simulink model "pv_and_batt"  (Simulink 7.8)
settings: Solver=ode45  StartTime=0.0  StopTime=10.0  RelTol=1e-3
values from neighbouring files (symbols this model uses):
  f = 60    [global_parameters.m]
  PLL_time_step = Ts    (= 8e-05)    [global_parameters.m]
  Td_es_min = Ts    (= 8e-05)    [global_parameters.m]
  Tds = Ts    (= 8e-05)    [global_parameters.m]
  Ts = 80e-6    (= 8e-05)    [global_parameters.m]    (also in scopeBuffer.m)
undefined symbols (not defined in the file or in its folder): batt_esr, C, D, DiscIntNeverNeededParam, I_ki, I_kp, Iac_max, Id_at_max, Iq_at_max, L, PLL_Ki, PLL_Kp, Roff, Vdc_max
libraries: powerlib x38, simulink x17, simulink_extras x6, cstextras x6, powerlib_extras x2, rtlab x1
(part 1 of 2)
settings Model: Creator=re25624  LastModifiedBy=ma25949

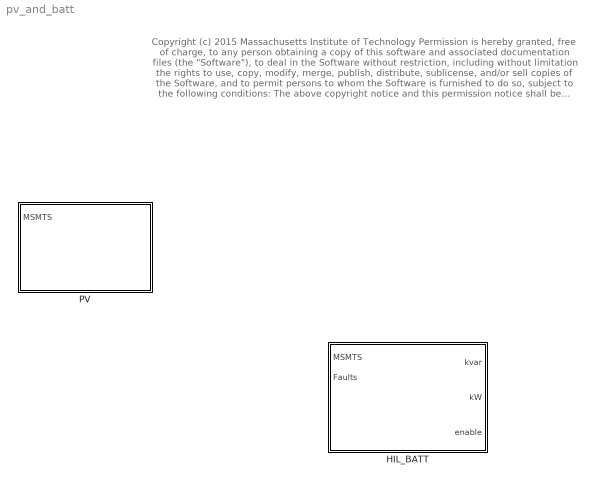
== system pv_and_batt ==
  note: Copyright (c) 2015 Massachusetts Institute of Technology
      | Permission is hereby granted, free of charge, to any person obtaining a copy of this software and associated documentation files (the "Software"), to deal in the Software without restriction, including without limitation the rights to use, copy, modify, merge, publish, distribute, sublicense, and/or sell copies of the Software, and to permit persons to whom the Software is furnished to do so, subject to the following conditions:
      |
      | The above copyright notice and this permission notice shall be included in all copies or substantial portions of the Software.
      |
      | THE SOFTWARE IS PROVIDED "AS IS", WITHOUT WARRANTY OF ANY KIND, EXPRESS OR IMPLIED, INCLUDING BUT NOT LIMITED TO THE WARRANTIES OF MERCHANTABILITY, FITNESS FOR A PARTICULAR PURPOSE AND NONINFRINGEMENT. IN NO EVENT SHALL THE AUTHORS OR COPYRIGHT HOLDERS BE LIABLE FOR ANY CLAIM,
      | DAMAGES OR OTHER LIABILITY, WHETHER IN AN ACTION OF CONTRACT, TORT OR OTHERWISE, ARISING FROM, OUT OF OR IN CONNECTION WITH THE SOFTWARE OR THE USE OR OTHER DEALINGS IN THE SOFTWARE.
  HIL_BATT : Subsystem
  PV : Subsystem

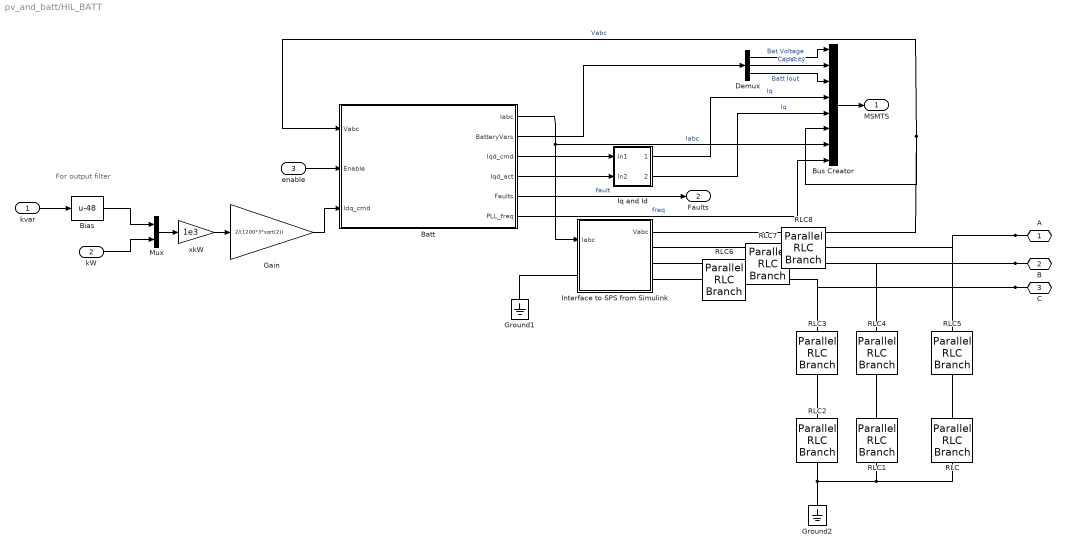
== system pv_and_batt/HIL_BATT ==
  note: For output filter
  kvar : Inport
  kW : Inport  Port=2
  enable : Inport  Port=3
  Batt : Subsystem  mask(Battery Energy Storage System with AC inverter and Droop Control){max_power=4e6, batt_kWh=5000, VacRMS=1200, Vdc_nom=4000}
      mask prompts: max_power "Peak Power (W)"; batt_kWh "Capacity (kWh)"; VacRMS "Grid Tie Line to Neutral Voltage (RMS)"; Vdc_nom "Nominal DC Battery Voltage"
      mask help: The block implements a battery energy storage system suitable for connecting to the grid. It responds to grid voltage changes by injecting current into the grid. The model is a non-switching average model.
      mask init:
      | global_parameters
      | BES_init
      mask Help:
      | This block will likely need a filter and transformer on it's output in order to connect to a high power line.
      | 
      | A unit delay block  on the Iabc output can help remove algebraic loops with minimal impact on simulation results.
      | 
      | 
      | Block Parameters:
      | Peak Power- Maximum power the unit can transfer.
      | Capacity- Amount of energy in the battery.
      | Grid Tie Line to Neutral Voltage- RMS voltage for the grid tie interface.
      | Nominal DC Battery Voltage- Open circuit full charge voltage.
      | Real Power Droop Gain- Ratio of Watts to Hz for injecting power to the grid in response to frequency changes.
      | Reactive Power Droop Gain- Ratio of kVars to RMS volts for injecting reactive power to the grid.
      | Droop Filter Cut Off- Fastest frequency that will be responded to for injecting power to the grid.
      | 
      | 
      | Block Connections:
      | Vabc- Grid voltage for each of the three phases.
      | Enable- Set to zero for no power.  Set to 1 to enable energy tranfer.
      | Iabc- Grid current for each of the three phases.  Connect to your grid.  Positive is into the grid.
      | Battery_vars- A vector of battery voltage, capacity, and current out of the battery.
      | Iqd_cmd- Commanded q and d axis currents.
      | Iqd_act- Actual q and d axis currents.
      mask Display:
      | image(imread('grid_storage_battery.jpg'))
      | color('white')
      | fprintf('%d kW Peak', max_power/1e3)
      | color('black')
      | port_label('input',1,'Vabc')
      | port_label('input',2,'Enable')
      | port_label('input',3,'Idq_cmd')
      | port_label('output',1,'Iabc')
      | port_label('output',2,'Battery_vars')
      | port_label('output',3,'Iqd_cmd')
      | port_label('output',4,'Iqd_act')
      | port_label('output',5,'Faults')
      | port_label('output',6,'Freq')
  Bias : Bias  Bias=-48
  Bus Creator : BusCreator  Inputs=8
  Demux : Demux  Outputs=3
  Gain : Gain  Gain=2/(1200*3*sqrt(2))
  Ground1 : powerlib/Elements/Ground  LConnTagsString=a
  Ground2 : powerlib/Elements/Ground  LConnTagsString=a
  Interface to SPS from Simulink : Subsystem
  Iq and Id : Subsystem
  Mux : Mux  Inputs=2
  "RLC " : powerlib/Elements/Parallel RLC Branch  LConnTagsString=a  RConnTagsString=__new0  BranchType=RLC  Resistance=500  Inductance=inf  SetiL0=off  InitialCurrent=0  Capacitance=10e-6  Setx0=off  InitialVoltage=0  Measurements=None
  RLC1 : powerlib/Elements/Parallel RLC Branch  LConnTagsString=a  RConnTagsString=__new0  BranchType=RLC  Resistance=500  Inductance=inf  SetiL0=off  InitialCurrent=0  Capacitance=10e-6  Setx0=off  InitialVoltage=0  Measurements=None
  RLC2 : powerlib/Elements/Parallel RLC Branch  LConnTagsString=a  RConnTagsString=__new0  BranchType=RLC  Resistance=500  Inductance=inf  SetiL0=off  InitialCurrent=0  Capacitance=10e-6  Setx0=off  InitialVoltage=0  Measurements=None
  RLC3 : powerlib/Elements/Parallel RLC Branch  LConnTagsString=a  RConnTagsString=__new0  BranchType=R  Resistance=10e-3  Inductance=inf  SetiL0=off  InitialCurrent=0  Capacitance=0  Setx0=off  InitialVoltage=0  Measurements=None
  RLC4 : powerlib/Elements/Parallel RLC Branch  LConnTagsString=a  RConnTagsString=__new0  BranchType=R  Resistance=10e-3  Inductance=inf  SetiL0=off  InitialCurrent=0  Capacitance=0  Setx0=off  InitialVoltage=0  Measurements=None
  RLC5 : powerlib/Elements/Parallel RLC Branch  LConnTagsString=a  RConnTagsString=__new0  BranchType=R  Resistance=10e-3  Inductance=inf  SetiL0=off  InitialCurrent=0  Capacitance=0  Setx0=off  InitialVoltage=0  Measurements=None
  RLC6 : powerlib/Elements/Parallel RLC Branch  LConnTagsString=a  RConnTagsString=__new0  BranchType=R  Resistance=20e-3  Inductance=inf  SetiL0=off  InitialCurrent=0  Capacitance=0  Setx0=off  InitialVoltage=0  Measurements=None
  RLC7 : powerlib/Elements/Parallel RLC Branch  LConnTagsString=a  RConnTagsString=__new0  BranchType=R  Resistance=20e-3  Inductance=inf  SetiL0=off  InitialCurrent=0  Capacitance=0  Setx0=off  InitialVoltage=0  Measurements=None
  RLC8 : powerlib/Elements/Parallel RLC Branch  LConnTagsString=a  RConnTagsString=__new0  BranchType=R  Resistance=20e-3  Inductance=inf  SetiL0=off  InitialCurrent=0  Capacitance=0  Setx0=off  InitialVoltage=0  Measurements=None
  xkW : Gain  Gain=1e3
  A : PMIOPort  Port=1  Side=Right
  B : PMIOPort  Port=2  Side=Right
  C : PMIOPort  Port=3  Side=Right
  MSMTS : Outport
  Faults : Outport  Port=2
  wires:
  Batt/5(Faults) -> Faults/1  "fault"
  Interface to SPS from Simulink/1(Vabc) -> Batt/1(Vabc), Bus Creator/6  "Vabc"
  Batt/2(BatteryVars) -> Demux/1
  Demux/2 -> Bus Creator/2  "Capacity"
  Demux/3 -> Bus Creator/3  "Batt Iout"
  Demux/1 -> Bus Creator/1  "Bat Voltage"
  Batt/3(Iqd_cmd) -> Iq and Id/1(In1)
  Batt/4(Iqd_act) -> Iq and Id/2(In2)
  Iq and Id/1(Out1) -> Bus Creator/4  "Iq"
  enable/1 -> Batt/2(Enable)
  Batt/1(Iabc) -> Bus Creator/7, Interface to SPS from Simulink/1(Iabc)  "Iabc"
  Gain/1 -> Batt/3(Idq_cmd)
  xkW/1 -> Gain/1
  Mux/1 -> xkW/1
  Iq and Id/2(Out2) -> Bus Creator/5  "Iq"
  Bus Creator/1 -> MSMTS/1
  kvar/1 -> Bias/1
  kW/1 -> Mux/2
  Batt/6(PLL_freq) -> Bus Creator/8  "freq"
  Bias/1 -> Mux/1
  connections:
  Interface to SPS from Simulink/LConn1 -- Ground1/LConn1
  Ground2/LConn1 -- RLC2/RConn1 -- "RLC "/RConn1 -- RLC1/RConn1
  A/RConn1 -- RLC8/LConn1 -- RLC5/LConn1
  B/RConn1 -- RLC7/LConn1 -- RLC4/LConn1
  C/RConn1 -- RLC6/LConn1 -- RLC3/LConn1
  RLC3/RConn1 -- RLC2/LConn1
  RLC4/RConn1 -- RLC1/LConn1
  RLC5/RConn1 -- "RLC "/LConn1
  RLC6/RConn1 -- Interface to SPS from Simulink/RConn3
  Interface to SPS from Simulink/RConn2 -- RLC7/RConn1
  Interface to SPS from Simulink/RConn1 -- RLC8/RConn1

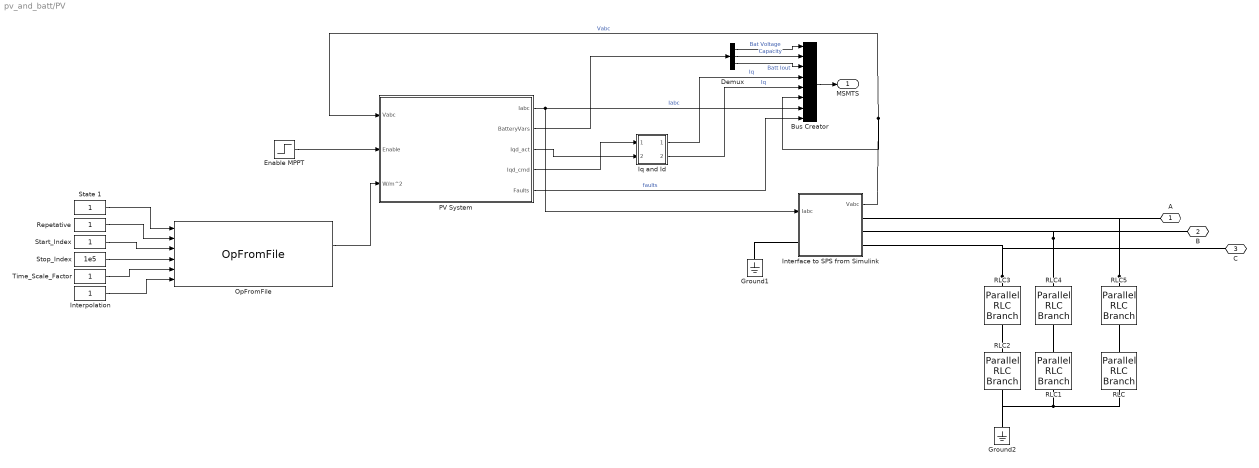
== system pv_and_batt/PV ==
  Bus Creator : BusCreator  Inputs=8
  Demux : Demux  Outputs=3
  Enable MPPT : Step  Time=0.5  SampleTime=Ts
  Ground1 : powerlib/Elements/Ground  LConnTagsString=a
  Ground2 : powerlib/Elements/Ground  LConnTagsString=a
  Interface to SPS from Simulink : Subsystem
  "Interpolation " : Constant
  Iq and Id : Subsystem
  OpFromFile : rtlab/DataLogging/OpFromFile  filename_mode=Static (same filename all the time)  reload_mode=Next time model is paused (Real-Time)  init_file_id=0  filename=irradiance_data.mat  rtpath='./'  nrtpath='.\'  sample_time=Ts
  PV System : Subsystem  mask(Battery Energy Storage System with AC inverter and Droop Control){max_power=4e6, VacRMS=1200, Vdc_nom=3500}
      mask prompts: max_power "Peak Power (W)"; VacRMS "Grid Tie Line to Neutral Voltage (RMS)"; Vdc_nom "Nominal DC Battery Voltage"
      mask help: The block implements a battery energy storage system suitable for connecting to the grid. It responds to grid voltage changes by injecting current into the grid. The model is a non-switching average model.
      mask init:
      | global_parameters
      | BES_init
      mask Help:
      | This block will likely need a filter and transformer on it's output in order to connect to a high power line.
      | 
      | A unit delay block  on the Iabc output can help remove algebraic loops with minimal impact on simulation results.
      | 
      | 
      | Block Parameters:
      | Peak Power- Maximum power the unit can transfer.
      | Capacity- Amount of energy in the battery.
      | Grid Tie Line to Neutral Voltage- RMS voltage for the grid tie interface.
      | Nominal DC Battery Voltage- Open circuit full charge voltage.
      | Real Power Droop Gain- Ratio of Watts to Hz for injecting power to the grid in response to frequency changes.
      | Reactive Power Droop Gain- Ratio of kVars to RMS volts for injecting reactive power to the grid.
      | Droop Filter Cut Off- Fastest frequency that will be responded to for injecting power to the grid.
      | 
      | 
      | Block Connections:
      | Vabc- Grid voltage for each of the three phases.
      | Enable- Set to zero for no power.  Set to 1 to enable energy tranfer.
      | Iabc- Grid current for each of the three phases.  Connect to your grid.  Positive is into the grid.
      | Battery_vars- A vector of battery voltage, capacity, and current out of the battery.
      | Iqd_cmd- Commanded q and d axis currents.
      | Iqd_act- Actual q and d axis currents.
  "RLC " : powerlib/Elements/Parallel RLC Branch  LConnTagsString=a  RConnTagsString=__new0  BranchType=RLC  Resistance=1e6  Inductance=inf  SetiL0=off  InitialCurrent=0  Capacitance=10e-6  Setx0=off  InitialVoltage=0  Measurements=None
  RLC1 : powerlib/Elements/Parallel RLC Branch  LConnTagsString=a  RConnTagsString=__new0  BranchType=RLC  Resistance=1e6  Inductance=inf  SetiL0=off  InitialCurrent=0  Capacitance=10e-6  Setx0=off  InitialVoltage=0  Measurements=None
  RLC2 : powerlib/Elements/Parallel RLC Branch  LConnTagsString=a  RConnTagsString=__new0  BranchType=RLC  Resistance=1e6  Inductance=inf  SetiL0=off  InitialCurrent=0  Capacitance=10e-6  Setx0=off  InitialVoltage=0  Measurements=None
  RLC3 : powerlib/Elements/Parallel RLC Branch  LConnTagsString=a  RConnTagsString=__new0  BranchType=R  Resistance=10e-3  Inductance=inf  SetiL0=off  InitialCurrent=0  Capacitance=0  Setx0=off  InitialVoltage=0  Measurements=None
  RLC4 : powerlib/Elements/Parallel RLC Branch  LConnTagsString=a  RConnTagsString=__new0  BranchType=R  Resistance=10e-3  Inductance=inf  SetiL0=off  InitialCurrent=0  Capacitance=0  Setx0=off  InitialVoltage=0  Measurements=None
  RLC5 : powerlib/Elements/Parallel RLC Branch  LConnTagsString=a  RConnTagsString=__new0  BranchType=R  Resistance=10e-3  Inductance=inf  SetiL0=off  InitialCurrent=0  Capacitance=0  Setx0=off  InitialVoltage=0  Measurements=None
  "Repetative " : Constant
  "Start_Index " : Constant
  State 1 : Constant
  "Stop_Index " : Constant  Value=1e5
  "Time_Scale_Factor " : Constant
  A : PMIOPort  Port=1  Side=Right
  B : PMIOPort  Port=2  Side=Right
  C : PMIOPort  Port=3  Side=Right
  MSMTS : Outport
  wires:
  PV System/4(Iqd_cmd) -> Iq and Id/1(In1)
  PV System/5(Faults) -> Bus Creator/8  "faults"
  Enable MPPT/1 -> PV System/2(Enable)
  Bus Creator/1 -> MSMTS/1
  Iq and Id/2(Out2) -> Bus Creator/5  "Iq"
  PV System/1(Iabc) -> Interface to SPS from Simulink/1(Iabc), Bus Creator/7  "Iabc"
  Iq and Id/1(Out1) -> Bus Creator/4  "Iq"
  PV System/3(Iqd_act) -> Iq and Id/2(In2)
  Demux/1 -> Bus Creator/1  "Bat Voltage"
  Demux/3 -> Bus Creator/3  "Batt Iout"
  Demux/2 -> Bus Creator/2  "Capacity"
  PV System/2(BatteryVars) -> Demux/1
  Interface to SPS from Simulink/1(Vabc) -> PV System/1(Vabc), Bus Creator/6  "Vabc"
  "Interpolation "/1 -> OpFromFile/6
  "Time_Scale_Factor "/1 -> OpFromFile/5
  "Stop_Index "/1 -> OpFromFile/4
  "Start_Index "/1 -> OpFromFile/3
  "Repetative "/1 -> OpFromFile/2
  State 1/1 -> OpFromFile/1
  OpFromFile/2 -> PV System/3(W/m^2)
  connections:
  "RLC "/LConn1 -- RLC5/RConn1
  RLC1/LConn1 -- RLC4/RConn1
  RLC3/RConn1 -- RLC2/LConn1
  RLC5/LConn1 -- A/RConn1 -- Interface to SPS from Simulink/RConn1
  RLC3/LConn1 -- C/RConn1 -- Interface to SPS from Simulink/RConn3
  Interface to SPS from Simulink/RConn2 -- B/RConn1 -- RLC4/LConn1
  RLC1/RConn1 -- "RLC "/RConn1 -- RLC2/RConn1 -- Ground2/LConn1
  Interface to SPS from Simulink/LConn1 -- Ground1/LConn1

== system pv_and_batt/HIL_BATT/Batt ==
  note: Positive current is into the DC bus.
  Vabc : Inport
  Enable : Inport  Port=2  OutDataTypeStr=double
  Idq_cmd : Inport  Port=3
  Battery : Subsystem  mask(Very simple battery model.  ){energy=batt_kWh, esr=batt_esr, Vdc_nom=Vdc_nom}
      mask prompts: energy "Capacity  (kWh)"; esr "Output Resistance (Ohms)"; Vdc_nom "Open Circuit Voltage"
      mask help: Model integrates charge and stops at the rated capacity. When charge is all removed the current drops to zero.
      mask Help: This model views the battery as a voltage source with a fixed equivalent series resistance and a perfect integrator for capacity.
  Data Type Conversion : DataTypeConversion  OutDataTypeStr=boolean
  Grid Tied Inverter : Subsystem
  Mux : Mux  Inputs=3
  Iabc : Outport
  BatteryVars : Outport  Port=2
  Iqd_cmd : Outport  Port=3
  Iqd_act : Outport  Port=4
  Faults : Outport  Port=5
  PLL_freq : Outport  Port=6
  wires:
  Data Type Conversion/1 -> Grid Tied Inverter/4(Enable)
  Enable/1 -> Data Type Conversion/1
  Idq_cmd/1 -> Iqd_cmd/1, Grid Tied Inverter/2(Iqd_ref)
  Grid Tied Inverter/4(Iqd) -> Iqd_act/1
  Mux/1 -> BatteryVars/1
  Grid Tied Inverter/1(Iabc) -> Iabc/1  "Iabc"
  Battery/2(Capacity) -> Mux/2  "Battery Capacity"
  Battery/1(Iout) -> Mux/3, Grid Tied Inverter/3(Idc)  "Iout Battery"
  Grid Tied Inverter/2(Vdc) -> Battery/1(Vout), Mux/1  "Vbat"
  Vabc/1 -> Grid Tied Inverter/1(Vabc)  "Vabc"
  Grid Tied Inverter/5(Faults) -> Faults/1
  Grid Tied Inverter/3(PLL_freq) -> PLL_freq/1

== system pv_and_batt/HIL_BATT/Interface to SPS from Simulink ==
  Iabc : Inport
  Controlled Current Source3 : powerlib/Electrical Sources/Controlled Current Source  Initialize=on  Source_Type=AC  Amplitude=0  Phase=0  Frequency=0  Measurements=None
  Controlled Current Source4 : powerlib/Electrical Sources/Controlled Current Source  Initialize=on  Source_Type=AC  Amplitude=0  Phase=0  Frequency=0  Measurements=None
  Controlled Current Source5 : powerlib/Electrical Sources/Controlled Current Source  Initialize=on  Source_Type=AC  Amplitude=0  Phase=0  Frequency=0  Measurements=None
  Demux4 : Demux  Outputs=3
  Gain : Gain  Gain=-1
  Mux2 : Mux  Inputs=3
  Voltage Measurement3 : powerlib/Measurements/Voltage Measurement  PhasorSimulation=off  OutputType=Complex  PSBequivalent=0
  Voltage Measurement4 : powerlib/Measurements/Voltage Measurement  PhasorSimulation=off  OutputType=Complex  PSBequivalent=0
  Voltage Measurement5 : powerlib/Measurements/Voltage Measurement  PhasorSimulation=off  OutputType=Complex  PSBequivalent=0
  Phase_A : PMIOPort  Port=1  Side=Right
  Phase_B : PMIOPort  Port=2  Side=Right
  Phase_C : PMIOPort  Port=3  Side=Right
  Ground : PMIOPort  Port=4  Side=Left
  Vabc : Outport
  wires:
  Gain/1 -> Demux4/1
  Voltage Measurement3/1 -> Mux2/1
  Mux2/1 -> Vabc/1
  Iabc/1 -> Gain/1
  Demux4/3 -> Controlled Current Source5/1
  Demux4/2 -> Controlled Current Source4/1
  Demux4/1 -> Controlled Current Source3/1
  Voltage Measurement4/1 -> Mux2/2
  Voltage Measurement5/1 -> Mux2/3
  connections:
  Phase_B/RConn1 -- Controlled Current Source4/RConn1 -- Voltage Measurement4/LConn1
  Ground/RConn1 -- Voltage Measurement5/LConn2 -- Voltage Measurement3/LConn2 -- Voltage Measurement4/LConn2 -- Controlled Current Source4/LConn1 -- Controlled Current Source3/LConn1 -- Controlled Current Source5/LConn1
  Phase_A/RConn1 -- Controlled Current Source3/RConn1 -- Voltage Measurement3/LConn1
  Phase_C/RConn1 -- Controlled Current Source5/RConn1 -- Voltage Measurement5/LConn1

== system pv_and_batt/HIL_BATT/Iq and Id ==
  In1 : Inport
  In2 : Inport  Port=2
  Demux1 : Demux  Outputs=2
  Demux2 : Demux  Outputs=2
  Mux : Mux  Inputs=2
  Mux1 : Mux  Inputs=2
  Out1 : Outport
  Out2 : Outport  Port=2
  wires:
  Demux1/2 -> Mux1/1  "Id_cmd"
  Demux2/1 -> Mux/2  "Iq_act"
  Demux1/1 -> Mux/1  "Iq_cmd"
  Demux2/2 -> Mux1/2  "Id_act"
  In1/1 -> Demux1/1
  In2/1 -> Demux2/1
  Mux/1 -> Out1/1
  Mux1/1 -> Out2/1

== system pv_and_batt/PV/Interface to SPS from Simulink ==
  Iabc : Inport
  Controlled Current Source3 : powerlib/Electrical Sources/Controlled Current Source  Initialize=on  Source_Type=AC  Amplitude=0  Phase=0  Frequency=0  Measurements=None
  Controlled Current Source4 : powerlib/Electrical Sources/Controlled Current Source  Initialize=on  Source_Type=AC  Amplitude=0  Phase=0  Frequency=0  Measurements=None
  Controlled Current Source5 : powerlib/Electrical Sources/Controlled Current Source  Initialize=on  Source_Type=AC  Amplitude=0  Phase=0  Frequency=0  Measurements=None
  Demux4 : Demux  Outputs=3
  Gain : Gain  Gain=-1
  Mux2 : Mux  Inputs=3
  Voltage Measurement3 : powerlib/Measurements/Voltage Measurement  PhasorSimulation=off  OutputType=Complex  PSBequivalent=0
  Voltage Measurement4 : powerlib/Measurements/Voltage Measurement  PhasorSimulation=off  OutputType=Complex  PSBequivalent=0
  Voltage Measurement5 : powerlib/Measurements/Voltage Measurement  PhasorSimulation=off  OutputType=Complex  PSBequivalent=0
  Phase_A : PMIOPort  Port=1  Side=Right
  Phase_B : PMIOPort  Port=2  Side=Right
  Phase_C : PMIOPort  Port=3  Side=Right
  Ground : PMIOPort  Port=4  Side=Left
  Vabc : Outport
  wires:
  Voltage Measurement5/1 -> Mux2/3
  Voltage Measurement4/1 -> Mux2/2
  Demux4/1 -> Controlled Current Source3/1
  Demux4/2 -> Controlled Current Source4/1
  Demux4/3 -> Controlled Current Source5/1
  Iabc/1 -> Gain/1
  Mux2/1 -> Vabc/1
  Voltage Measurement3/1 -> Mux2/1
  Gain/1 -> Demux4/1
  connections:
  Voltage Measurement5/LConn1 -- Controlled Current Source5/RConn1 -- Phase_C/RConn1
  Voltage Measurement3/LConn1 -- Controlled Current Source3/RConn1 -- Phase_A/RConn1
  Controlled Current Source5/LConn1 -- Controlled Current Source3/LConn1 -- Controlled Current Source4/LConn1 -- Voltage Measurement4/LConn2 -- Voltage Measurement3/LConn2 -- Voltage Measurement5/LConn2 -- Ground/RConn1
  Voltage Measurement4/LConn1 -- Controlled Current Source4/RConn1 -- Phase_B/RConn1

== system pv_and_batt/PV/Iq and Id ==
  In1 : Inport
  In2 : Inport  Port=2
  Demux1 : Demux  Outputs=2
  Demux2 : Demux  Outputs=2
  Mux : Mux  Inputs=2
  Mux1 : Mux  Inputs=2
  Out1 : Outport
  Out2 : Outport  Port=2
  wires:
  Mux1/1 -> Out2/1
  Mux/1 -> Out1/1
  In2/1 -> Demux2/1
  In1/1 -> Demux1/1
  Demux2/2 -> Mux1/2  "Id_act"
  Demux1/1 -> Mux/1  "Iq_cmd"
  Demux2/1 -> Mux/2  "Iq_act"
  Demux1/2 -> Mux1/1  "Id_cmd"

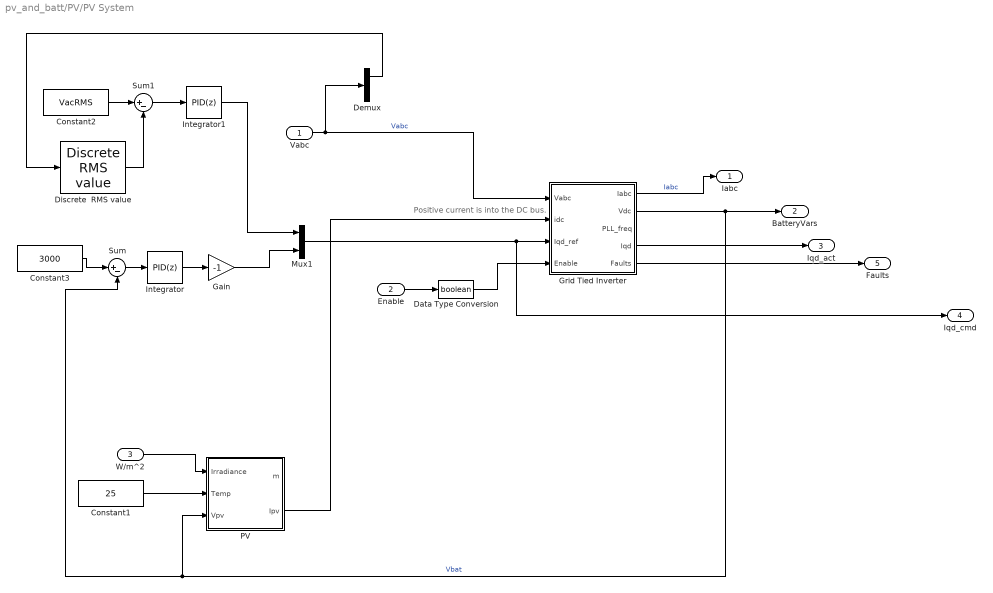
== system pv_and_batt/PV/PV System ==
  note: Positive current is into the DC bus.
  Vabc : Inport
  Enable : Inport  Port=2  OutDataTypeStr=double
  W/m^2 : Inport  Port=3
  Constant1 : Constant  Value=25
  Constant2 : Constant  Value=VacRMS
  Constant3 : Constant  Value=3000
  Data Type Conversion : DataTypeConversion  OutDataTypeStr=boolean
  Demux : Demux  Outputs=3
  Discrete  RMS value : powerlib_extras/Discrete Measurements/Discrete  RMS value  Freq=60  Mag_Init=1200  Ts=50e-6
  Gain : Gain  Gain=-1
  Grid Tied Inverter : Subsystem
  Integrator : simulink/Continuous/PID Controller  Controller=PID  TimeDomain=Discrete-time  SampleTime=Ts  IntegratorMethod=Forward Euler  FilterMethod=Forward Euler  Form=Parallel  P=4  I=3  D=0  N=100  InitialConditionSource=internal  InitialConditionForIntegrator=0  InitialConditionForFilter=0  ExternalReset=none  LimitOutput=on  UpperSaturationLimit=2000  LowerSaturationLimit=-2000  LinearizeAsGain=off  AntiWindupMode=clamping  Kb=1  TrackingMode=off  Kt=1  PParamMin=[]  PParamMax=[]  IParamMin=[]  IParamMax=[]  DParamMin=[]  DParamMax=[]  NParamMin=[]  NParamMax=[]  KbParamMin=[]  KbParamMax=[]  KtParamMin=[]  KtParamMax=[]  POutMin=[]  POutMax=[]  IOutMin=[]  IOutMax=[]  DOutMin=[]  DOutMax=[]  NOutMin=[]  NOutMax=[]  KbOutMin=[]  KbOutMax=[]  KtOutMin=[]  KtOutMax=[]  IntegratorOutMin=[]  IntegratorOutMax=[]  FilterOutMin=[]  FilterOutMax=[]  SumOutMin=[]  SumOutMax=[]  SumI1OutMin=[]  SumI1OutMax=[]  SumI2OutMin=[]  SumI2OutMax=[]  SumI3OutMin=[]  SumI3OutMax=[]  SumDOutMin=[]  SumDOutMax=[]  SaturationOutMin=[]  SaturationOutMax=[]  IntegratorContinuousStateAttributes=''  IntegratorStateMustResolveToSignalObject=off  IntegratorRTWStateStorageClass=Auto  FilterContinuousStateAttributes=''  FilterStateMustResolveToSignalObject=off  FilterRTWStateStorageClass=Auto
  Integrator1 : simulink/Continuous/PID Controller  Controller=PID  TimeDomain=Discrete-time  SampleTime=Ts  IntegratorMethod=Forward Euler  FilterMethod=Forward Euler  Form=Parallel  P=4  I=3  D=0  N=100  InitialConditionSource=internal  InitialConditionForIntegrator=0  InitialConditionForFilter=0  ExternalReset=none  LimitOutput=on  UpperSaturationLimit=2000  LowerSaturationLimit=-2000  LinearizeAsGain=off  AntiWindupMode=clamping  Kb=1  TrackingMode=off  Kt=1  PParamMin=[]  PParamMax=[]  IParamMin=[]  IParamMax=[]  DParamMin=[]  DParamMax=[]  NParamMin=[]  NParamMax=[]  KbParamMin=[]  KbParamMax=[]  KtParamMin=[]  KtParamMax=[]  POutMin=[]  POutMax=[]  IOutMin=[]  IOutMax=[]  DOutMin=[]  DOutMax=[]  NOutMin=[]  NOutMax=[]  KbOutMin=[]  KbOutMax=[]  KtOutMin=[]  KtOutMax=[]  IntegratorOutMin=[]  IntegratorOutMax=[]  FilterOutMin=[]  FilterOutMax=[]  SumOutMin=[]  SumOutMax=[]  SumI1OutMin=[]  SumI1OutMax=[]  SumI2OutMin=[]  SumI2OutMax=[]  SumI3OutMin=[]  SumI3OutMax=[]  SumDOutMin=[]  SumDOutMax=[]  SaturationOutMin=[]  SaturationOutMax=[]  IntegratorContinuousStateAttributes=''  IntegratorStateMustResolveToSignalObject=off  IntegratorRTWStateStorageClass=Auto  FilterContinuousStateAttributes=''  FilterStateMustResolveToSignalObject=off  FilterRTWStateStorageClass=Auto
  Mux1 : Mux  Inputs=2
  PV : Subsystem  mask{Ncell=60, Nser=102, Npar=158, Voc_Tref=38, Isc_Tref=8.9, Eg=1.12, dVdI_Voc=-0.32, K0=0.05, Rs=0.349, Rsh=111.55, IL=8.944, Vm=30.5, Im=8.03, PlotVI_module=off, PlotVI_array=off}
      mask prompts: Ncell "Number of cells per module"; Nser "Number of series-connected module per string"; Npar "Numer of parallel strings"; Voc_Tref "Open circuit voltage Voc (V)"; Isc_Tref "Short circuit current Isc (A)"; Eg "Band gap energy of crystalline silicon (eV)"; dVdI_Voc "Temperature coefficient of Voc (%/C)"; K0 "Temperature coefficient of Isc (%/C)"; Rs "Series resistance Rs (Ohms)"; Rsh "Shunt resistance Rsh (Ohms)"; IL "Light-generated current IL (A)"; Vm "Maximum Power Point Voltage Vmpp (V)"; Im "Maximum Powe Point Current Impp (A)"; PlotVI_module "Display  I-V and  P-V characteritics of one module"; PlotVI_array "Display  I-V and  P-V characteritics of array"
      mask init:
      | BlockName=gcb;
      | 
      | 
      | q = 1.6022e-19; % electron charge
      | k = 1.3806e-23; % Boltzman constant
      | n = 1.55; % diode quality factor
      | Tref_K = 273.15+25; % 25C to K
      | Gnom = 1000; % nominal irradiation in W/m^2
      | VT_ref = Ncell*n*k*Tref_K/q; 
      | I0_Tref = Isc_Tref/(exp(Voc_Tref/VT_ref)-1);
      | % Xv = I0_Tref*q*exp(Voc_Tref/VT_ref)/n/k/Tref_K;
      | % Rs = -dVdI_Voc-1/Xv; 
      | 
      | %% Plot I-V & P-V characteristics of one module
      | %==============================================
      | if PlotVI_module | PlotVI_array
      |     assignin('base','Voc_Tref',Voc_Tref);
      |     assignin('base','Isc_Tref',Isc_Tref);
      |     assignin('base','Rs',Rs);
      |     assignin('base','Rsh',Rsh);
      |     assignin('base','I0_Tref',I0_Tref);
      |     assignin('base','VT_ref',VT_ref);
      |      
      |     if PlotVI_module, 
      |         F1 = figure('Name','I-V characteristics of one module at 25 deg.C');
      |         F2 = figure('Name','P-V characteristics of one module at 25 deg.C');
      |     end
      |     if PlotVI_array ,
      |         F3 = figure('Name','I-V characteristics of array at 25 deg.C'); 
      |         F4 = figure('Name','P-V characteristics of array at 25 deg.C'); 
      |     end
      |     load_system('PV_param_plot_model');
      |     
      |     for ksun = 1:-0.2:0.2
      |         assignin('base','IL',IL*ksun)
      |         sim('PV_param_plot_model');
      |         n = find(I_PV >= 0);
      |         I_PV = I_PV(n);
      |         V_PV = V_PV(n);
      |         P_PV = V_PV.*I_PV;
      |         
      |         if PlotVI_module
      |             figure(F1);
      |             if ksun == 1
      |                 
      |                 plot(V_PV,I_PV,'b')
      |                % plot(V_PV,I_PV,'b',[0  Vm Voc_Tref], [Isc_Tref Im 0],'ro')
      |                 text(Voc_Tref/15,Isc_Tref*1.1,'1 kW/m^2')
      |                 hold on
      |                 grid
      |             else
      |                 plot(V_PV,I_PV,'--m')
      |                 text(Voc_Tref/15, Isc_Tref*(ksun+0.1) , sprintf('%g kW/m^2',ksun))
      |             end
      | 
      |             figure(F2); 
      |             if ksun == 1
      |                 
      |                 plot(V_PV,I_PV,'b')
      |                 %plot(V_PV,P_PV,'b',[0  Vm Voc_Tref], [0 Im*Vm 0],'ro')
      |                 text(Vm*1.02,Vm*Im,'1 kW/m^2')
      |                 hold on
      |                 grid
      |             else
      |                 n = find(P_PV == max(P_PV));
      |                 % plot(V_PV,P_PV,'--m', V_PV(n) , P_PV(n),'mo')
      |                 plot(V_PV,P_PV,'--m')
      |                 text(Vm*1.02, Vm*Im*ksun, sprintf('%g kW/m^2',ksun))
      |             end
      |             figure(F1); 
      |             ylabel('Current (A)')
      |             xlabel('Voltage (V)')
      |             axis_xy = axis;
      |             axis_xy(4) = Isc_Tref*1.2;
      |             axis(axis_xy);
      |             
      |             figure(F2);
      |             ylabel('Power (W)')
      |             xlabel('Voltage (V)')
      |             axis_xy = axis;
      |             axis_xy(4) = Vm*Im*1.2;
      |             axis(axis_xy);
      |                   
      |             set_param(BlockName,'PlotVI_module', 'off')
      |         end
      |         
      |         if PlotVI_array
      |             figure(F3);
      |             if ksun == 1
      |                 plot(V_PV*Nser,I_PV*Npar,'b')
      |                 % plot(V_PV*Nser,I_PV*Npar,'b',[0  Vm Voc_Tref]*Nser, [Isc_Tref Im 0]*Npar,'ro')
      |                 text(Voc_Tref/15*Nser,Isc_Tref*1.1*Npar,'1 kW/m^2')
      |                 hold on
      |                 grid
      |             else
      |                 plot(V_PV*Nser,I_PV*Npar,'--m')
      |                 text(Voc_Tref*Nser/15, Isc_Tref*Npar*(ksun+0.1) , sprintf('%g kW/m^2',ksun))
      |             end
      |            
      | 
      |             figure(F4);
      |             if ksun == 1
      |                 plot(V_PV*Nser,P_PV*Nser*Npar,'b')
      |                 % plot(V_PV*Nser,P_PV*Nser*Npar,'b',[0  Vm Voc_Tref]*Nser, [0 Im*Vm 0]*Nser*Npar,'ro')
      |                 text(Vm*Nser*1.02,Vm*Im*Nser*Npar,'1 kW/m^2')
      |                 hold on
      |                 grid
      |             else
      |                 n = find(P_PV == max(P_PV));
      |                 plot(V_PV*Nser,P_PV*Nser*Npar,'--m')
      |                 % plot(V_PV*Nser,P_PV*Nser*Npar,'--m', V_PV(n)*Nser , P_PV(n)*Nser*Npar,'mo')
      |                 text(Vm*Nser*1.02, Vm*Im*Nser*Npar*ksun, sprintf('%g kW/m^2',ksun))
      |             end 
      |             figure(F3);
      |             ylabel('Current (A)')
      |             xlabel('Voltage (V)')
      |             axis_xy = axis;
      |             axis_xy(4) = Isc_Tref*Npar*1.2;
      |             axis(axis_xy);
      |             
      |             figure(F4);
      |             ylabel('Power (W)')
      |             xlabel('Voltage (V)')
      |             xis_xy = axis;
      |             axis_xy(4) = Vm*Im*Nser*Npar*1.2;
      |             axis(axis_xy);
      |             
      |             set_param(BlockName,'PlotVI_array', 'off')
      |         end
      |         
      |     end  
      | end
  Sum : Sum  Inputs=|+-
  Sum1 : Sum  Inputs=|+-
  Iabc : Outport
  BatteryVars : Outport  Port=2
  Iqd_act : Outport  Port=3
  Iqd_cmd : Outport  Port=4
  Faults : Outport  Port=5
  wires:
  Data Type Conversion/1 -> Grid Tied Inverter/4(Enable)
  Enable/1 -> Data Type Conversion/1
  Grid Tied Inverter/4(Iqd) -> Iqd_act/1
  Grid Tied Inverter/1(Iabc) -> Iabc/1  "Iabc"
  Grid Tied Inverter/2(Vdc) -> BatteryVars/1, PV/3(Vpv), Sum/2  "Vbat"
  Vabc/1 -> Grid Tied Inverter/1(Vabc), Demux/1  "Vabc"
  W/m^2/1 -> PV/1(Irradiance)
  Constant1/1 -> PV/2(Temp)
  PV/2(Ipv) -> Grid Tied Inverter/2(idc)
  Mux1/1 -> Grid Tied Inverter/3(Iqd_ref), Iqd_cmd/1
  Sum/1 -> Integrator/1
  Integrator/1 -> Gain/1
  Constant3/1 -> Sum/1
  Gain/1 -> Mux1/2
  Integrator1/1 -> Mux1/1
  Sum1/1 -> Integrator1/1
  Constant2/1 -> Sum1/1
  Discrete  RMS value/1 -> Sum1/2
  Demux/1 -> Discrete  RMS value/1
  Grid Tied Inverter/5(Faults) -> Faults/1

== system pv_and_batt/HIL_BATT/Batt/Battery ==
  note: An attempt was made to reduce the rate at which this block
      | needs to be calculated with 1ms rate transition on
      | Vout .  It greatly improved calc time but it caused instability.
  Vout : Inport
  Add : Sum  Inputs=-+
  Compare To Constant : simulink/Logic and Bit Operations/Compare To Constant  relop=>  const=0  OutDataTypeStr=uint8
  Constant : Constant  Value=Vdc_nom  SampleTime=Tds
  Discrete-Time Integrator : DiscreteIntegrator  InitialCondition=energy*3600*0.5  InitialConditionMode=State only (most efficient)  SampleTime=Tds  LimitOutput=on  UpperSaturationLimit=energy*3600  LowerSaturationLimit=0  ICPrevOutput=DiscIntNeverNeededParam  ICPrevScaledInput=DiscIntNeverNeededParam
  Gain1 : Gain  Gain=-Vdc_nom/3600
  Gain2 : Gain  Gain=1/(energy*3600)
  IC : InitialCondition  Value=Vdc_nom
  IC1 : InitialCondition  Value=0
  Mult : Product  Inputs=**
  RT6 : RateTransition  OutPortSampleTime=Tds
  Resr : Gain  Gain=-1/esr
  Iout : Outport
  Capacity : Outport  Port=2
  wires:
  RT6/1 -> Mult/2
  IC1/1 -> Iout/1
  IC/1 -> Add/2
  Discrete-Time Integrator/1 -> Gain2/1
  Gain2/1 -> Compare To Constant/1, Capacity/1
  Resr/1 -> Gain1/1, RT6/1
  Mult/1 -> IC1/1
  Vout/1 -> IC/1
  Compare To Constant/1 -> Mult/1
  Gain1/1 -> Discrete-Time Integrator/1
  Add/1 -> Resr/1
  Constant/1 -> Add/1

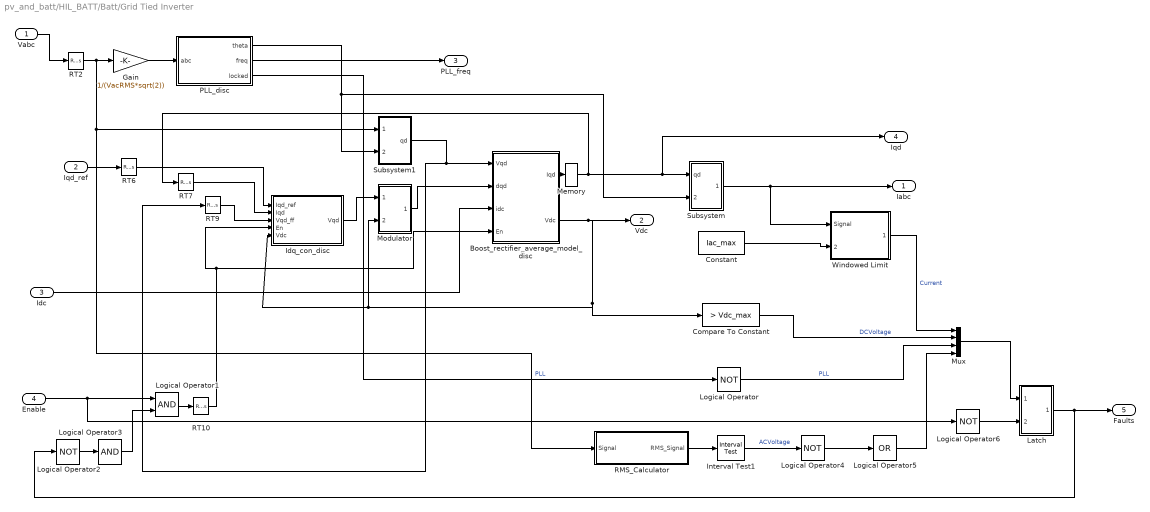
== system pv_and_batt/HIL_BATT/Batt/Grid Tied Inverter ==
  Vabc : Inport
  Iqd_ref : Inport  Port=2
  Idc : Inport  Port=3
  Enable : Inport  Port=4
  Boost_rectifier_average_model_disc : Subsystem  mask{C=C, L=L, Roff=Roff, Vdc_nom=Vdc_nom}
      mask prompts: C "DC Bus Capacitance"; L "Boost Inductor"; Roff "Switch resistance when off"; Vdc_nom "Nominal DC Bus Voltage"
      mask init:
      | global_parameters
  Compare To Constant : simulink/Logic and Bit Operations/Compare To Constant  relop=>  const=Vdc_max  OutDataTypeStr=boolean
  Constant : Constant  Value=Iac_max
  Gain : Gain  Gain=1/(VacRMS*sqrt(2))
  Idq_con_disc : Subsystem  mask{L=L, iq_max=Iq_at_max, id_max=Id_at_max, kp=I_kp, ki=I_ki, Vdc_nom=Vdc_nom}
      mask prompts: L "Boost Inductor"; iq_max "Maximum Iq"; id_max "Maximum Id"; kp "Proportional Gain"; ki "Integral Gain"; Vdc_nom "Nominal DC Bus Voltage"
      mask init:
      | global_parameters
  Interval Test1 : simulink/Logic and Bit Operations/Interval Test  IntervalClosedRight=on  uplimit=VacRMS*1.1  IntervalClosedLeft=on  lowlimit=VacRMS*0.9  OutDataTypeStr=boolean
  Latch : Subsystem
  Logical Operator{,2,4,6} (4 alike) : Logic  Operator=NOT  AllPortsSameDT=off  OutDataTypeStr=boolean
  Logical Operator1 : Logic  AllPortsSameDT=off  OutDataTypeStr=boolean
  Logical Operator3 : Logic  Inputs=1  AllPortsSameDT=off  OutDataTypeStr=boolean
  Logical Operator5 : Logic  Operator=OR  Inputs=1  AllPortsSameDT=off  OutDataTypeStr=boolean
  Memory : Memory  InheritSampleTime=on
  Modulator : Subsystem
  Mux : Mux
  PLL_disc : Subsystem  mask{PLL_Kp=PLL_Kp, PLL_Ki=PLL_Ki, PLL_freq_range=0.25, PLL_lock_window=0.1}
      mask prompts: PLL_Kp "Proportional Gain"; PLL_Ki "Integral Gain"; PLL_freq_range "PLL Frequency Range"; PLL_lock_window "PLL Lock Window"
  RMS_Calculator : Subsystem
  RT{2,6..7,9..10} (5 alike) : RateTransition  OutPortSampleTime=Td_es_min
  Subsystem : Subsystem
  Subsystem1 : Subsystem
  Windowed Limit : Subsystem
  Iabc : Outport
  Vdc : Outport  Port=2
  PLL_freq : Outport  Port=3
  Iqd : Outport  Port=4
  Faults : Outport  Port=5
  wires:
  Memory/1 -> RT7/1, Iqd/1, Subsystem/1(qd)
  RT10/1 -> Idq_con_disc/4(En), Boost_rectifier_average_model_disc/4(En)
  RT9/1 -> Idq_con_disc/3(Vqd_ff)
  RT6/1 -> Idq_con_disc/1(Iqd_ref)
  RT2/1 -> Gain/1, Subsystem1/1(abc), RMS_Calculator/1(Signal)
  Vabc/1 -> RT2/1
  PLL_disc/1(theta) -> Subsystem/2(theta), Subsystem1/2(theta)
  Enable/1 -> Logical Operator1/1, Logical Operator6/1
  Gain/1 -> PLL_disc/1(abc)
  Logical Operator/1 -> Mux/3  "PLL"
  PLL_disc/3(locked) -> Logical Operator/1  "PLL"
  Modulator/1(dqd) -> Boost_rectifier_average_model_disc/2(dqd)
  PLL_disc/2(freq) -> PLL_freq/1
  Compare To Constant/1 -> Mux/2  "DCVoltage"
  Windowed Limit/1(TestOut) -> Mux/1  "Current"
  Constant/1 -> Windowed Limit/2(Threshold)
  Logical Operator1/1 -> RT10/1
  Idq_con_disc/1(Vqd) -> Modulator/1(Vqd)
  Iqd_ref/1 -> RT6/1
  Subsystem/1(abc) -> Iabc/1, Windowed Limit/1(Signal)
  Boost_rectifier_average_model_disc/1(Iqd) -> Memory/1
  Subsystem1/1(qd) -> Boost_rectifier_average_model_disc/1(Vqd), RT9/1
  Logical Operator2/1 -> Logical Operator3/1
  Logical Operator3/1 -> Logical Operator1/2
  RMS_Calculator/1(RMS_Signal) -> Interval Test1/1
  Interval Test1/1 -> Logical Operator4/1  "ACVoltage"
  Logical Operator4/1 -> Logical Operator5/1
  Logical Operator5/1 -> Mux/4
  Boost_rectifier_average_model_disc/2(Vdc) -> Vdc/1, Idq_con_disc/5(Vdc), Modulator/2(Vdc), Compare To Constant/1
  Idc/1 -> Boost_rectifier_average_model_disc/3(idc)
  RT7/1 -> Idq_con_disc/2(Iqd)
  Mux/1 -> Latch/1(In1)
  Logical Operator6/1 -> Latch/2(Reset)
  Latch/1(Out1) -> Logical Operator2/1, Faults/1

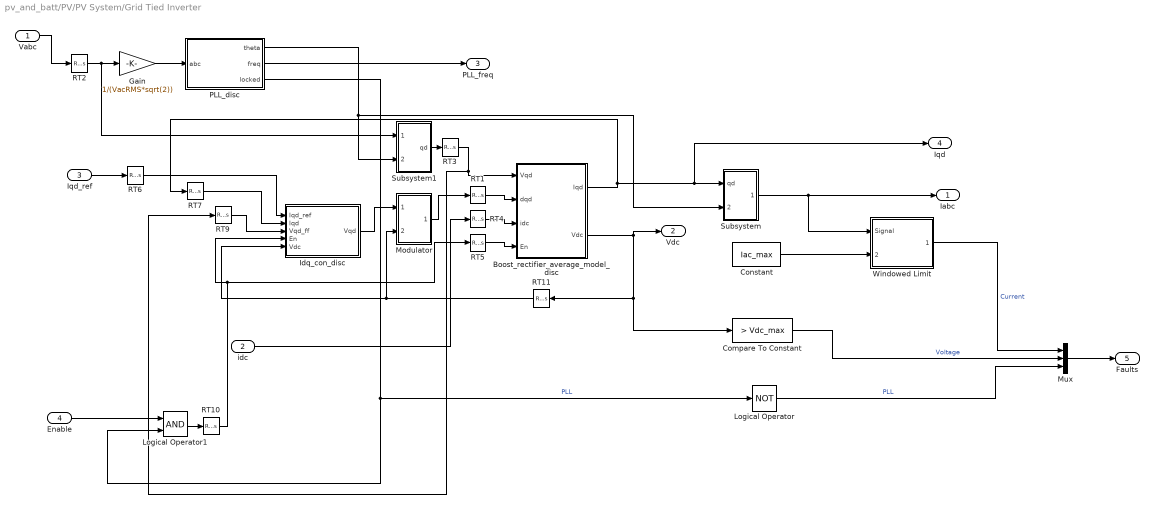
== system pv_and_batt/PV/PV System/Grid Tied Inverter ==
  Vabc : Inport
  idc : Inport  Port=2
  Iqd_ref : Inport  Port=3
  Enable : Inport  Port=4
  Boost_rectifier_average_model_disc : Subsystem  mask{C=C, L=L, Roff=Roff, Vdc_nom=Vdc_nom}
      mask prompts: C "DC Bus Capacitance"; L "Boost Inductor"; Roff "Switch resistance when off"; Vdc_nom "Nominal DC Bus Voltage"
      mask init:
      | global_parameters
  Compare To Constant : simulink/Logic and Bit Operations/Compare To Constant  relop=>  const=Vdc_max  OutDataTypeStr=boolean
  Constant : Constant  Value=Iac_max
  Gain : Gain  Gain=1/(VacRMS*sqrt(2))
  Idq_con_disc : Subsystem  mask{L=L, iq_max=Iq_at_max, id_max=Id_at_max*2, kp=I_kp, ki=I_ki, Vdc_nom=Vdc_nom}
      mask prompts: L "Boost Inductor"; iq_max "Maximum Iq"; id_max "Maximum Id"; kp "Proportional Gain"; ki "Integral Gain"; Vdc_nom "Nominal DC Bus Voltage"
      mask init:
      | global_parameters
  Logical Operator : Logic  Operator=NOT  AllPortsSameDT=off  OutDataTypeStr=boolean
  Logical Operator1 : Logic  AllPortsSameDT=off  OutDataTypeStr=boolean
  Modulator : Subsystem
  Mux : Mux  Inputs=3
  PLL_disc : Subsystem  mask{PLL_Kp=PLL_Kp, PLL_Ki=PLL_Ki, PLL_freq_range=0.25, PLL_lock_window=0.1}
      mask prompts: PLL_Kp "Proportional Gain"; PLL_Ki "Integral Gain"; PLL_freq_range "PLL Frequency Range"; PLL_lock_window "PLL Lock Window"
  RT{1,3..5} (4 alike) : RateTransition
  RT{2,6..7,9..11} (6 alike) : RateTransition  OutPortSampleTime=Td_es_min
  Subsystem : Subsystem
  Subsystem1 : Subsystem
  Windowed Limit : Subsystem
  Iabc : Outport
  Vdc : Outport  Port=2
  PLL_freq : Outport  Port=3
  Iqd : Outport  Port=4
  Faults : Outport  Port=5
  wires:
  RT11/1 -> Modulator/2(Vdc), Idq_con_disc/5(Vdc)
  RT10/1 -> RT5/1, Idq_con_disc/4(En)
  RT9/1 -> Idq_con_disc/3(Vqd_ff)
  Boost_rectifier_average_model_disc/2(Vdc) -> Compare To Constant/1, RT11/1, Vdc/1
  RT7/1 -> Idq_con_disc/2(Iqd)
  RT6/1 -> Idq_con_disc/1(Iqd_ref)
  RT5/1 -> Boost_rectifier_average_model_disc/4(En)
  RT4/1 -> Boost_rectifier_average_model_disc/3(idc)
  RT3/1 -> RT9/1, Boost_rectifier_average_model_disc/1(Vqd)
  RT2/1 -> Subsystem1/1(abc), Gain/1
  Vabc/1 -> RT2/1
  RT1/1 -> Boost_rectifier_average_model_disc/2(dqd)
  PLL_disc/1(theta) -> Subsystem1/2(theta), Subsystem/2(theta)
  Enable/1 -> Logical Operator1/1
  Gain/1 -> PLL_disc/1(abc)
  Logical Operator/1 -> Mux/3  "PLL"
  PLL_disc/3(locked) -> Logical Operator1/2, Logical Operator/1  "PLL"
  Modulator/1(dqd) -> RT1/1
  PLL_disc/2(freq) -> PLL_freq/1
  Compare To Constant/1 -> Mux/2  "Voltage"
  Windowed Limit/1(TestOut) -> Mux/1  "Current"
  Constant/1 -> Windowed Limit/2(Threshold)
  Logical Operator1/1 -> RT10/1
  idc/1 -> RT4/1
  Idq_con_disc/1(Vqd) -> Modulator/1(Vqd)
  Iqd_ref/1 -> RT6/1
  Subsystem/1(abc) -> Iabc/1, Windowed Limit/1(Signal)
  Boost_rectifier_average_model_disc/1(Iqd) -> RT7/1, Iqd/1, Subsystem/1(qd)
  Subsystem1/1(qd) -> RT3/1
  Mux/1 -> Faults/1

== system pv_and_batt/PV/PV System/PV ==
  Irradiance : Inport
  Temp : Inport  Port=2
  Vpv : Inport  Port=3
  Bus Creator : BusCreator  Inputs=5
  Controlled Voltage Source : powerlib/Electrical Sources/Controlled Voltage Source  Initialize=on  Source_Type=DC  Amplitude=1200  Phase=0  Frequency=0  Measurements=None
  Diode : Subsystem
      mask Display:
      | plot(-75,-50,100,150, [-15 -15 43 -15 -15 -75],[50 8 50 92 50 50], ...
      |     [43 43],[8 94],[100 43], [50 50])
  Gain1 : Gain  Gain=Rs*Nser/Npar  SaturateOnIntegerOverflow=on  OutDataTypeStr=Inherit: Same as input  ParamDataTypeStr=Inherit: Same as input
  IL : powerlib/Electrical Sources/Controlled Current Source  Initialize=on  Source_Type=AC  Amplitude=0  Phase=0  Frequency=0  Measurements=None
  I_PV : powerlib/Measurements/Current Measurement  PhasorSimulation=off  OutputType=Complex  PSBequivalent=0
  Light current IL : Subsystem
  Product : Product  RndMeth=Zero
  Rs : powerlib/Elements/Series RLC Branch  LConnTagsString=__new0  RConnTagsString=__new0  BranchType=R  Resistance=Rs*Nser/Npar  Inductance=1e-3  SetiL0=off  InitialCurrent=0  Capacitance=1e-6  Setx0=off  InitialVoltage=0  Measurements=None
  Rsh : powerlib/Elements/Series RLC Branch  LConnTagsString=__new0  RConnTagsString=__new0  BranchType=R  Resistance=Rsh*Nser/Npar  Inductance=1e-3  SetiL0=off  InitialCurrent=0  Capacitance=1e-6  Setx0=off  InitialVoltage=0  Measurements=Branch current
  Sum2 : Sum  SaturateOnIntegerOverflow=on  InputSameDT=on  OutDataTypeStr=Inherit: Same as first input
  V_PV : powerlib/Measurements/Voltage Measurement  PhasorSimulation=off  OutputType=Complex  PSBequivalent=0
  m : Outport
  Ipv : Outport  Port=2
  wires:
  Product/1 -> Bus Creator/3  "P_PV"
  Bus Creator/1 -> m/1
  Temp/1 -> Bus Creator/4, Light current IL/1(Temperature)  "Temperature (C)"
  Gain1/1 -> Sum2/1
  Sum2/1 -> Diode/1(Vd)
  I_PV/1 -> Product/2, Bus Creator/2, Gain1/1, Ipv/1  "I_PV"
  V_PV/1 -> Product/1, Bus Creator/1, Sum2/2  "V_PV"
  Light current IL/1(IL) -> IL/1
  Irradiance/1 -> Bus Creator/5, Light current IL/2(Irradiance)  "Irradiance (W/m^2)"
  Vpv/1 -> Controlled Voltage Source/1
  Light current IL/2(Tcell_K) -> Diode/2(Tcell_K)
  connections:
  Controlled Voltage Source/RConn1 -- I_PV/RConn1 -- V_PV/LConn1
  Rs/LConn1 -- I_PV/LConn1
  Diode/RConn1 -- IL/LConn1 -- Rsh/RConn1 -- Controlled Voltage Source/LConn1 -- V_PV/LConn2
  Rs/RConn1 -- IL/RConn1 -- Diode/LConn1 -- Rsh/LConn1

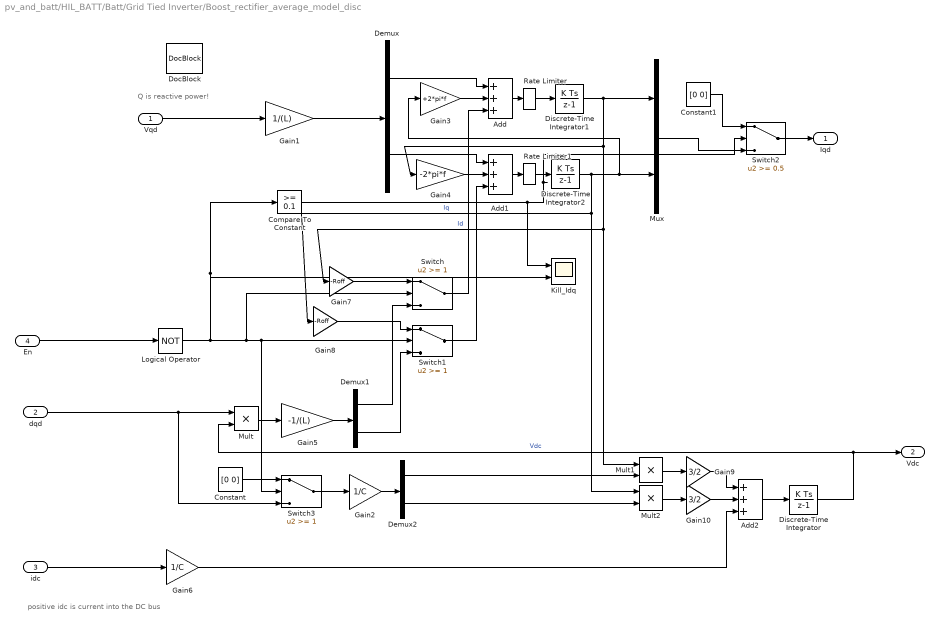
== system pv_and_batt/HIL_BATT/Batt/Grid Tied Inverter/Boost_rectifier_average_model_disc ==
  note: Q is reactive power!
  note: positive idc is current into the DC bus
  Vqd : Inport
  dqd : Inport  Port=2  PortDimensions=2
  idc : Inport  Port=3
  En : Inport  Port=4  OutDataTypeStr=boolean
  Add : Sum  Inputs=+++
  Add1 : Sum  Inputs=+++
  Add2 : Sum  Inputs=+++
  Compare To Constant : simulink/Logic and Bit Operations/Compare To Constant  relop=>=  const=0.1  OutDataTypeStr=uint8
  Constant : Constant  Value=[0 0]
  Constant1 : Constant  Value=[0 0]
  Demux : Demux  Outputs=2
  Demux1 : Demux  Outputs=2
  Demux2 : Demux  Outputs=2
  Discrete-Time Integrator : DiscreteIntegrator  InitialCondition=Vdc_nom  InitialConditionMode=State only (most efficient)  SampleTime=Tds  ICPrevOutput=DiscIntNeverNeededParam  ICPrevScaledInput=DiscIntNeverNeededParam
  Discrete-Time Integrator1 : DiscreteIntegrator  InitialConditionMode=State only (most efficient)  SampleTime=Tds  ICPrevOutput=DiscIntNeverNeededParam  ICPrevScaledInput=DiscIntNeverNeededParam
  Discrete-Time Integrator2 : DiscreteIntegrator  InitialConditionMode=State only (most efficient)  SampleTime=Tds  ICPrevOutput=DiscIntNeverNeededParam  ICPrevScaledInput=DiscIntNeverNeededParam
  DocBlock : simulink/Model-Wide Utilities/DocBlock  DocumentType=Text
  Gain1 : Gain  Gain=1/(L)
  Gain10 : Gain  Gain=3/2
  Gain2 : Gain  Gain=1/C
  Gain3 : Gain  Gain=+2*pi*f
  Gain4 : Gain  Gain=-2*pi*f
  Gain5 : Gain  Gain=-1/(L)
  Gain6 : Gain  Gain=1/C
  Gain7 : Gain  Gain=-Roff
  Gain8 : Gain  Gain=-Roff
  Gain9 : Gain  Gain=3/2
  Kill_Idq : Scope  NumInputPorts=2
      settings: YMin=-1~0.95  YMax=1~1.05  SaveName=ScopeData17
  Logical Operator : Logic  Operator=NOT  AllPortsSameDT=off  OutDataTypeStr=boolean
  Mult : Product  Inputs=**
  Mult1 : Product  Inputs=**
  Mult2 : Product  Inputs=**
  Mux : Mux  Inputs=2
  Rate Limiter : RateLimiter  RisingSlewLimit=1e6  FallingSlewLimit=-1e6  SampleTimeMode=inherited
  Rate Limiter1 : RateLimiter  RisingSlewLimit=1e6  FallingSlewLimit=-1e6  SampleTimeMode=inherited
  Switch : Switch  Threshold=1
  Switch1 : Switch  Threshold=1
  Switch2 : Switch  Threshold=0.5
  Switch3 : Switch  Threshold=1
  Iqd : Outport
  Vdc : Outport  Port=2
  wires:
  Rate Limiter1/1 -> Discrete-Time Integrator2/1
  Rate Limiter/1 -> Discrete-Time Integrator1/1
  Add1/1 -> Rate Limiter1/1
  Gain8/1 -> Switch1/1
  Discrete-Time Integrator2/1 -> Mux/2, Gain3/1, Mult2/1, Gain8/1  "Iq"
  Demux1/2 -> Switch1/3
  Mult1/1 -> Gain9/1
  Switch1/1 -> Add1/3
  Add/1 -> Rate Limiter/1
  Switch/1 -> Add/3
  Gain1/1 -> Demux/1
  Gain5/1 -> Demux1/1
  Mult2/1 -> Gain10/1
  Constant/1 -> Switch3/1
  Gain9/1 -> Add2/1
  Demux2/2 -> Mult2/2
  idc/1 -> Gain6/1
  Mult/1 -> Gain5/1
  Add2/1 -> Discrete-Time Integrator/1
  Gain7/1 -> Switch/1
  Demux/1 -> Add/1
  En/1 -> Logical Operator/1
  Discrete-Time Integrator1/1 -> Mux/1, Gain4/1, Mult1/1, Gain7/1  "Id"
  Switch3/1 -> Gain2/1
  Logical Operator/1 -> Switch/2, Switch1/2, Switch3/2, Compare To Constant/1, Kill_Idq/2
  Gain10/1 -> Add2/2
  Gain6/1 -> Add2/3
  Gain2/1 -> Demux2/1
  Demux1/1 -> Switch/3
  Gain4/1 -> Add1/2
  Gain3/1 -> Add/2
  Demux2/1 -> Mult1/2
  Demux/2 -> Add1/1
  Discrete-Time Integrator/1 -> Vdc/1, Mult/2  "Vdc"
  dqd/1 -> Mult/1, Switch3/3
  Vqd/1 -> Gain1/1
  Compare To Constant/1 -> Switch2/2, Kill_Idq/1
  Switch2/1 -> Iqd/1
  Constant1/1 -> Switch2/1
  Mux/1 -> Switch2/3

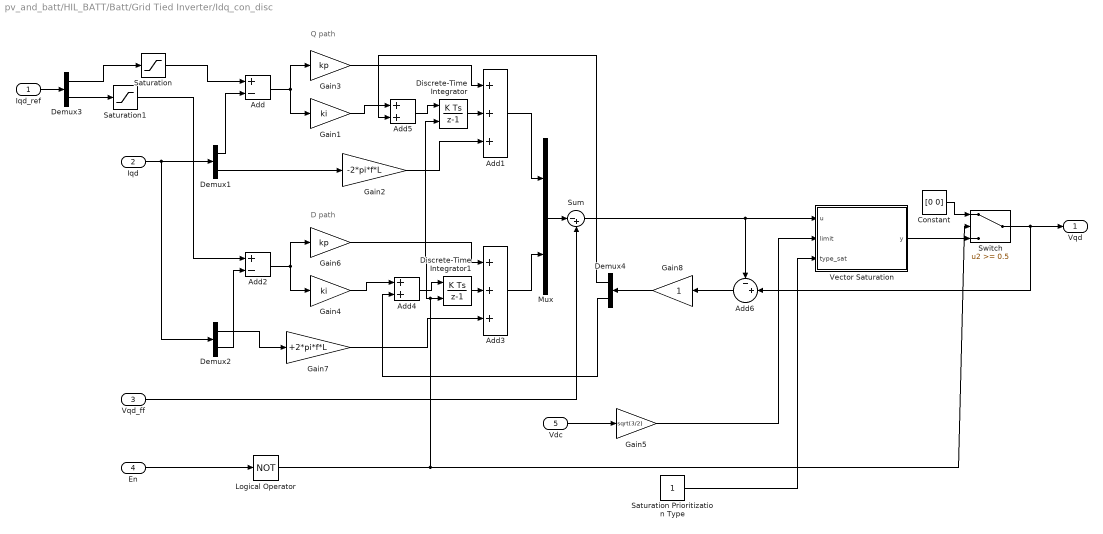
== system pv_and_batt/HIL_BATT/Batt/Grid Tied Inverter/Idq_con_disc ==
  note: Q path
  note: D path
  Iqd_ref : Inport
  Iqd : Inport  Port=2
  Vqd_ff : Inport  Port=3  PortDimensions=2
  En : Inport  Port=4  OutDataTypeStr=boolean  PortDimensions=1
  Vdc : Inport  Port=5  PortDimensions=1
  Add : Sum  Inputs=+-
  Add1 : Sum  Inputs=+++
  Add2 : Sum  Inputs=+-
  Add3 : Sum  Inputs=+++
  Add4 : Sum
  Add5 : Sum
  Add6 : Sum  Inputs=-+|
  Constant : Constant  Value=[0 0]
  Demux{1..4} (4 alike) : Demux  Outputs=2
  Discrete-Time Integrator : DiscreteIntegrator  ExternalReset=level  InitialConditionMode=State only (most efficient)  SampleTime=Td_es_min  ICPrevOutput=DiscIntNeverNeededParam  ICPrevScaledInput=DiscIntNeverNeededParam
  Discrete-Time Integrator1 : DiscreteIntegrator  ExternalReset=level  InitialConditionMode=State only (most efficient)  SampleTime=Td_es_min  ICPrevOutput=DiscIntNeverNeededParam  ICPrevScaledInput=DiscIntNeverNeededParam
  Gain1 : Gain  Gain=ki
  Gain2 : Gain  Gain=-2*pi*f*L
  Gain3 : Gain  Gain=kp
  Gain4 : Gain  Gain=ki
  Gain5 : Gain  Gain=sqrt(3/2)
  Gain6 : Gain  Gain=kp
  Gain7 : Gain  Gain=+2*pi*f*L
  Gain8 : Gain
  Logical Operator : Logic  Operator=NOT  AllPortsSameDT=off  OutDataTypeStr=boolean
  Mux : Mux  Inputs=2
  Saturation : Saturate  UpperLimit=iq_max  LowerLimit=-iq_max
  Saturation Prioritization Type : Constant
  Saturation1 : Saturate  UpperLimit=id_max  LowerLimit=-id_max
  Sum : Sum  Inputs=|-+
  Switch : Switch  Threshold=0.5
  Vector Saturation : MATLAB Function  TreatAsAtomicUnit=on
  Vqd : Outport
  wires:
  Add/1 -> Gain1/1, Gain3/1
  Gain6/1 -> Add3/1
  Demux4/2 -> Add4/2
  Mux/1 -> Sum/1
  Discrete-Time Integrator1/1 -> Add3/2
  Gain7/1 -> Add3/3
  Demux2/2 -> Add2/2
  Add3/1 -> Mux/2
  En/1 -> Logical Operator/1
  Gain1/1 -> Add5/1
  Gain2/1 -> Add1/3
  Demux3/2 -> Saturation1/1
  Discrete-Time Integrator/1 -> Add1/2
  Iqd/1 -> Demux2/1, Demux1/1
  Add4/1 -> Discrete-Time Integrator1/1
  Demux3/1 -> Saturation/1
  Add5/1 -> Discrete-Time Integrator/1
  Gain4/1 -> Add4/1
  Add1/1 -> Mux/1
  Sum/1 -> Vector Saturation/1(u), Add6/1
  Gain3/1 -> Add1/1
  Demux1/1 -> Add/2
  Demux1/2 -> Gain2/1
  Add2/1 -> Gain4/1, Gain6/1
  Gain8/1 -> Demux4/1
  Iqd_ref/1 -> Demux3/1
  Saturation1/1 -> Add2/1
  Saturation/1 -> Add/1
  Demux4/1 -> Add5/2
  Demux2/1 -> Gain7/1
  Vqd_ff/1 -> Sum/2
  Saturation Prioritization Type/1 -> Vector Saturation/3(type_sat)
  Gain5/1 -> Vector Saturation/2(limit)
  Add6/1 -> Gain8/1
  Vdc/1 -> Gain5/1
  Switch/1 -> Vqd/1, Add6/2
  Logical Operator/1 -> Discrete-Time Integrator/2, Discrete-Time Integrator1/2, Switch/2
  Vector Saturation/1(y) -> Switch/3
  Constant/1 -> Switch/1

== system pv_and_batt/HIL_BATT/Batt/Grid Tied Inverter/Latch ==
  In1 : Inport
  Reset : Inport  Port=2
  Demux : Demux  Outputs=6
  Mux : Mux  Inputs=6
  S-R Flip-Flop{,1..5} (6 alike) : simulink_extras/Flip Flops/S-R Flip-Flop  initial_condition=0
  Out1 : Outport
  wires:
  Reset/1 -> S-R Flip-Flop1/2, S-R Flip-Flop/2, S-R Flip-Flop2/2, S-R Flip-Flop3/2, S-R Flip-Flop4/2, S-R Flip-Flop5/2
  Demux/2 -> S-R Flip-Flop1/1
  S-R Flip-Flop1/1 -> Mux/2  "Ib"
  In1/1 -> Demux/1
  Demux/1 -> S-R Flip-Flop/1
  Mux/1 -> Out1/1  "Faults"
  S-R Flip-Flop/1 -> Mux/1  "Ia"
  S-R Flip-Flop2/1 -> Mux/3  "Ic"
  Demux/3 -> S-R Flip-Flop2/1
  Demux/4 -> S-R Flip-Flop3/1
  Demux/5 -> S-R Flip-Flop4/1
  Demux/6 -> S-R Flip-Flop5/1
  S-R Flip-Flop3/1 -> Mux/4  "Vdc"
  S-R Flip-Flop4/1 -> Mux/5  "PLL"
  S-R Flip-Flop5/1 -> Mux/6  "Vac"

== system pv_and_batt/HIL_BATT/Batt/Grid Tied Inverter/Modulator ==
  Vqd : Inport
  Vdc : Inport  Port=2
  Delay : Delay  DelayLength=1  InitialCondition=[0 0]  SampleTime=Td_es_min
  IC : InitialCondition  Value=Vdc_nom
  Mult1 : Product  Inputs=*/
  Saturation : Saturate  UpperLimit=1  LowerLimit=-1
  dqd : Outport
  wires:
  Delay/1 -> dqd/1
  IC/1 -> Mult1/2
  Vdc/1 -> IC/1
  Vqd/1 -> Mult1/1
  Saturation/1 -> Delay/1
  Mult1/1 -> Saturation/1
